simulink model "full_vehicle_sim"  (R2025b)
settings: Solver=VariableStepAuto  StartTime=0.0  StopTime=5  RelTol=1e-3
libraries: SimscapeFluids_lib x9, fl_lib x7, nesl_utility x5
(part 1 of 3)
settings Model: Creator=Owner  LastModifiedBy=25han
settings OptimizationCC: ReuseModelBlockBuffer=off
settings RTWCC: GPUComputeCapability=3.5

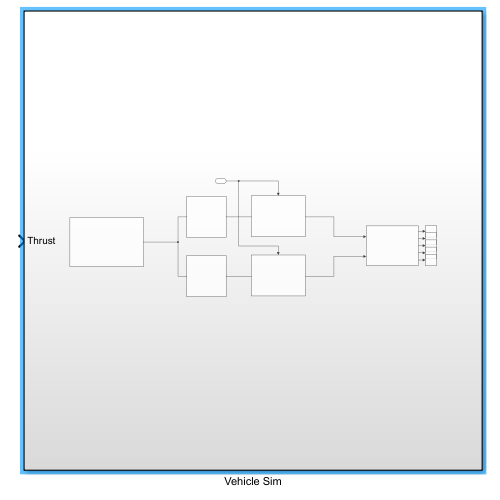
[thumbnail: Simulink's stored preview of the top-level diagram]
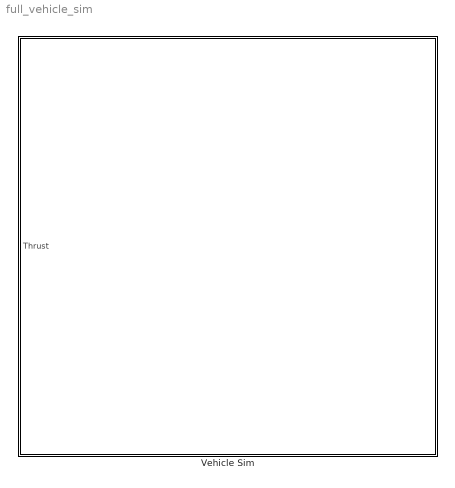
== system full_vehicle_sim ==
  Vehicle Sim : Subsystem

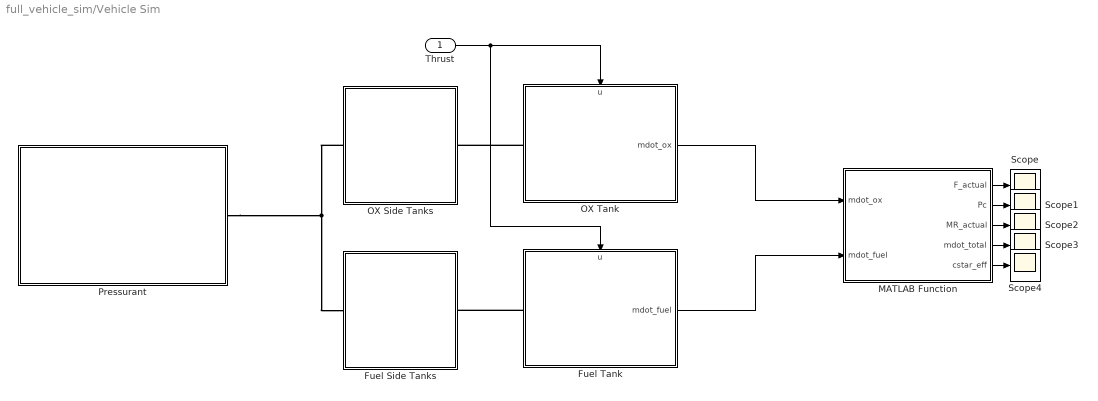
== system full_vehicle_sim/Vehicle Sim ==
  Thrust : Inport
  Fuel Side Tanks : Subsystem
  Fuel Tank : Subsystem
      settings: PortSchema="{\"entries\":[{\"content\":{\"sides\":[{\"content\":{\"connectorIds\":[\"LConn1\"]},\"type\":\"ConnectorPlacement.EquallySpacedRectSide\",\"uuid\":\"c996b4f4-0c8e-4748-a91d-4f7536df207c\"},{\"content\":{\"connectorIds\":[\"Out1\"],\"side\":\"RIGHT\"},\"type\":\"ConnectorPlacement.EquallySpacedRectSide\",\"uuid\":\"73da1da1-fc22-4773-8903-2723ce6ce475\"},{\"content\":{\"connectorIds\":[\"In1\"],\"side\":\"TOP\"},\"type\":\"ConnectorPlacement.EquallySpacedRectSide\",\"uuid\":\"cc756c5a-3437-4588-9c13-c05ccaf9d8e8\"}]},\"type\":\"ConnectorPlacement.EquallySpacedConnector\",\"uuid\":\"5391969f-ee8c-4c4c-8257-59a80b6e733b\"}],\"packageUris\":[\"http://schema.mathworks.com/mf0/Connector/R2020b\"],\"version\":\"1.0\"}"
  MATLAB Function : MATLAB Function  TreatAsAtomicUnit=on
  OX Side Tanks : Subsystem
  OX Tank : Subsystem
      settings: PortSchema="{\"entries\":[{\"content\":{\"sides\":[{\"content\":{\"connectorIds\":[\"LConn1\"]},\"type\":\"ConnectorPlacement.EquallySpacedRectSide\",\"uuid\":\"c996b4f4-0c8e-4748-a91d-4f7536df207c\"},{\"content\":{\"connectorIds\":[\"Out1\"],\"side\":\"RIGHT\"},\"type\":\"ConnectorPlacement.EquallySpacedRectSide\",\"uuid\":\"73da1da1-fc22-4773-8903-2723ce6ce475\"},{\"content\":{\"connectorIds\":[\"In1\"],\"side\":\"TOP\"},\"type\":\"ConnectorPlacement.EquallySpacedRectSide\",\"uuid\":\"cc756c5a-3437-4588-9c13-c05ccaf9d8e8\"}]},\"type\":\"ConnectorPlacement.EquallySpacedConnector\",\"uuid\":\"5391969f-ee8c-4c4c-8257-59a80b6e733b\"}],\"packageUris\":[\"http://schema.mathworks.com/mf0/Connector/R2020b\"],\"version\":\"1.0\"}"
  Pressurant : Subsystem
  Scope{,1..4} (5 alike) : Scope
      Scope settings: DataLoggingVariableName=ScopeData6
      Scope1 settings: DataLoggingVariableName=ScopeData7
      Scope2 settings: DataLoggingVariableName=ScopeData8
      Scope3 settings: DataLoggingVariableName=ScopeData9
      Scope4 settings: DataLoggingVariableName=ScopeData10
  wires:
  Thrust/1 -> OX Tank/1(u), Fuel Tank/1(u)
  Fuel Tank/1(mdot_fuel) -> MATLAB Function/2(mdot_fuel)
  OX Tank/1(mdot_ox) -> MATLAB Function/1(mdot_ox)
  MATLAB Function/2(Pc) -> Scope1/1
  MATLAB Function/3(MR_actual) -> Scope2/1
  MATLAB Function/4(mdot_total) -> Scope3/1
  MATLAB Function/5(cstar_eff) -> Scope4/1
  MATLAB Function/1(F_actual) -> Scope/1
  connections:
  OX Side Tanks/LConn1 -- Pressurant/RConn1 -- Fuel Side Tanks/LConn1
  OX Tank/LConn1 -- OX Side Tanks/RConn1
  Fuel Tank/LConn1 -- Fuel Side Tanks/RConn1

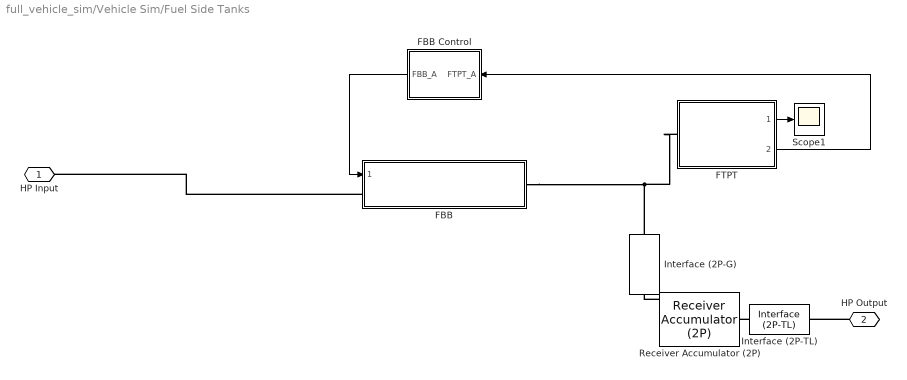
== system full_vehicle_sim/Vehicle Sim/Fuel Side Tanks ==
  FBB : Subsystem  ReferencedSubsystem=BangBang
  FBB Control : MATLAB Function  TreatAsAtomicUnit=on
  FTPT : Subsystem  ReferencedSubsystem=PT  max_press=5000  lower_val=4  upper_val=20
  Interface (2P-G) : SimscapeFluids_lib/Fluid Network Interfaces/Interface (2P-G)  area=0.01 m^2  vapor_error_spec=simscape.enum.assert.action.error
      settings: InternalSimscapePortConfiguration="{\"Bottom\":[],\"Left\":[{\"id\":\"x2P\",\"label\":\"2P\",\"type\":\"foundation.two_phase_fluid.two_phase_fluid\"}],\"Right\":[{\"id\":\"G\",\"label\":\"G\",\"type\":\"foundation.gas.gas\"}],\"Top\":[]}"
  Interface (2P-TL) : SimscapeFluids_lib/Fluid Network Interfaces/Interface (2P-TL)  area=0.01 m^2  liquid_error_spec=simscape.enum.assert.action.error
      settings: InternalSimscapePortConfiguration="{\"Bottom\":[],\"Left\":[{\"id\":\"x2P\",\"label\":\"2P\",\"type\":\"foundation.two_phase_fluid.two_phase_fluid\"}],\"Right\":[{\"id\":\"TL\",\"label\":\"TL\",\"type\":\"foundation.thermal_liquid.thermal_liquid\"}],\"Top\":[]}"
  Receiver Accumulator (2P) : SimscapeFluids_lib/Two-Phase Fluid/Tanks & Accumulators/Receiver Accumulator (2P)  volume=1 m^3  tank_area=0.5 m^2  area_AV=0.01 m^2  area_BV=0.01 m^2  area_AL=0.01 m^2  area_BL=0.01 m^2  V_frac_liq_error=simscape.enum.assert.action.none  V_frac_liq_min=0.05  V_frac_liq_max=0.95  V_frac_smooth=0.05  p_crit_error=simscape.enum.assert.action.error  hc_vap=20 W/(K*m^2)  hc_liq=100 W/(K*m^2)  p_init=0.101325 MPa  fraction_spec=fluids.two_phase_fluid.tanks_accumulators.enum.LiquidFractionSpec.Volume  M_frac_liq_init=0.5  V_frac_liq_init=0.5  saturated_init=true  energy_spec=fluids.two_phase_fluid.tanks_accumulators.enum.EnergySpec.SubcoolingSuperheating  delta_T_sub_init=5 deltaK  delta_T_sup_init=5 deltaK  T_liq_init=368.15 K  T_vap_init=378.15 K  h_liq_init=400 kJ/kg  h_vap_init=2700 kJ/kg  u_liq_init=400 kJ/kg  u_vap_init=2700 kJ/kg  tau_vap_cond=0.1 s
      settings: InternalSimscapePortConfiguration="{\"Bottom\":[],\"Left\":[{\"id\":\"AV\",\"label\":\"AV\",\"type\":\"foundation.two_phase_fluid.two_phase_fluid\"},{\"id\":\"AL\",\"label\":\"AL\",\"type\":\"foundation.two_phase_fluid.two_phase_fluid\"},{\"id\":\"H\",\"label\":\"H\",\"type\":\"foundation.thermal.thermal\"}],\"Right\":[{\"id\":\"BV\",\"label\":\"BV\",\"type\":\"foundation.two_phase_fluid.two_phase_fluid\"},{\"id\":\"BL\",\"label\":\"BL\",\"type\":\"foundation.two_phase_fluid.two_phase_fluid\"},{\"id\":\"L\",\"label\":\"L\",\"type\":\"output\"}],\"Top\":[]}"
  Scope1 : Scope
      settings: ActiveDisplayYMinimum=-330.96571  ActiveDisplayYMaximum=5077.33873
  HP Input : PMIOPort  Side=Left
  HP Output : PMIOPort  Port=2  Side=Right
  wires:
  FTPT/1 -> Scope1/1
  FTPT/2 -> FBB Control/1(FTPT_A)
  FBB Control/1(FBB_A) -> FBB/1
  connections:
  FBB/LConn1 -- HP Input/RConn1
  FTPT/LConn1 -- Interface (2P-G)/RConn1 -- FBB/RConn1
  Receiver Accumulator (2P)/LConn1 -- Interface (2P-G)/LConn1
  HP Output/RConn1 -- Interface (2P-TL)/RConn1
  Interface (2P-TL)/LConn1 -- Receiver Accumulator (2P)/RConn2

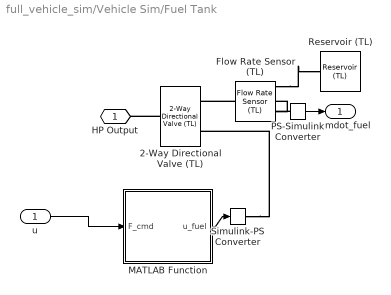
== system full_vehicle_sim/Vehicle Sim/Fuel Tank ==
  u : Inport
  2-Way Directional Valve (TL) : SimscapeFluids_lib/Thermal Liquid/Valves & Orifices/Directional Control Valves/2-Way Directional Valve (TL)  valve_spec=fluids.thermal_liquid.valves.directional_control_valves.enum.ValveSpec.Linear  S_max=5e-3 m  del_S_max=5e-3 m  area_max=1e-4 m^2  area_leak=1e-10 m^2  del_S_TLU=[0, .002, .004, .007, .017] m  valve_area_TLU=[1e-09, 2.0352e-07, 4.0736e-05, .00011438, .00034356] m^2  del_S_flow_TLU=[0, .002, .004, .007, .017] m  p_diff_TLU=[.3, .5, .7] MPa  vol_flow_TLU=1e-3 * [1.7e-05, 2e-05, 2.6e-05; .0035, .0045, .0053; .7, .9, 1.06; 1.96, 2.5, 3; 6, 7.7, 9.13] m^3/s  mdot_TLU=[1.7e-05, 2e-05, 2.6e-05; .0035, .0045, .0053; .7, .9, 1.06; 1.96, 2.5, 3; 6, 7.7, 9.13] kg/s  T_ref_in=293.15 K  p_ref_in=0.101325 MPa  Cd=0.64  Re_c=150  smoothing_factor=0.01  pressure_recovery=false  area=0.01 m^2
      settings: InternalSimscapePortConfiguration="{\"Bottom\":[],\"Left\":[{\"id\":\"A\",\"label\":\"A\",\"type\":\"foundation.thermal_liquid.thermal_liquid\"}],\"Right\":[{\"id\":\"S\",\"label\":\"S\",\"type\":\"input\"},{\"id\":\"B\",\"label\":\"B\",\"type\":\"foundation.thermal_liquid.thermal_liquid\"}],\"Top\":[]}"
  Flow Rate Sensor (TL) : fl_lib/Thermal Liquid/Sensors/Flow Rate Sensor (TL)  mass_flow_measure=true  volumetric_flow_measure=false  energy_flow_measure=true
      settings: InternalSimscapePortConfiguration="{\"Bottom\":[{\"id\":\"PHI\",\"label\":\"φ\",\"type\":\"output\"}],\"Left\":[{\"id\":\"A\",\"label\":\"A\",\"type\":\"foundation.thermal_liquid.thermal_liquid\"}],\"Right\":[{\"id\":\"B\",\"label\":\"B\",\"type\":\"foundation.thermal_liquid.thermal_liquid\"},{\"id\":\"M\",\"label\":\"M\",\"type\":\"output\"}],\"Top\":[]}"
  MATLAB Function : MATLAB Function  TreatAsAtomicUnit=on
  PS-Simulink Converter : nesl_utility/PS-Simulink Converter  PhysicalDomain=network_engine_domain  SubClassName=ps_output  LeftPortType=input  RightPortType=output  PseudoPeriodic=off  Frequencies=[]  VectorFormat=inherit  Unit=inherit  AffineConversion=off
  Reservoir (TL) : fl_lib/Thermal Liquid/Elements/Reservoir (TL)  pressure_spec=foundation.enum.pressure_spec.atmospheric  reservoir_pressure=0.101325 MPa  reservoir_temperature=293.15 K  area=0.01 m^2
  Simulink-PS Converter : nesl_utility/Simulink-PS Converter  PhysicalDomain=network_engine_domain  SubClassName=ps_input  LeftPortType=input  RightPortType=output  PseudoPeriodic=off  Frequencies=[]  NoiseDistribution=none  NoiseParameters=[]  Unit=1  AffineConversion=off  FilteringAndDerivatives=provide  SimscapeFilterOrder=1  InputFilterTimeConstant=0.001  UdotUserProvided=0
  HP Output : PMIOPort  Side=Left
  mdot_fuel : Outport
  wires:
  u/1 -> MATLAB Function/1(F_cmd)
  MATLAB Function/1(u_fuel) -> Simulink-PS Converter/1
  PS-Simulink Converter/1 -> mdot_fuel/1
  connections:
  2-Way Directional Valve (TL)/LConn1 -- HP Output/RConn1
  Flow Rate Sensor (TL)/LConn1 -- 2-Way Directional Valve (TL)/RConn2
  Simulink-PS Converter/RConn1 -- 2-Way Directional Valve (TL)/RConn1
  PS-Simulink Converter/LConn1 -- Flow Rate Sensor (TL)/RConn2
  Flow Rate Sensor (TL)/RConn1 -- Reservoir (TL)/LConn1

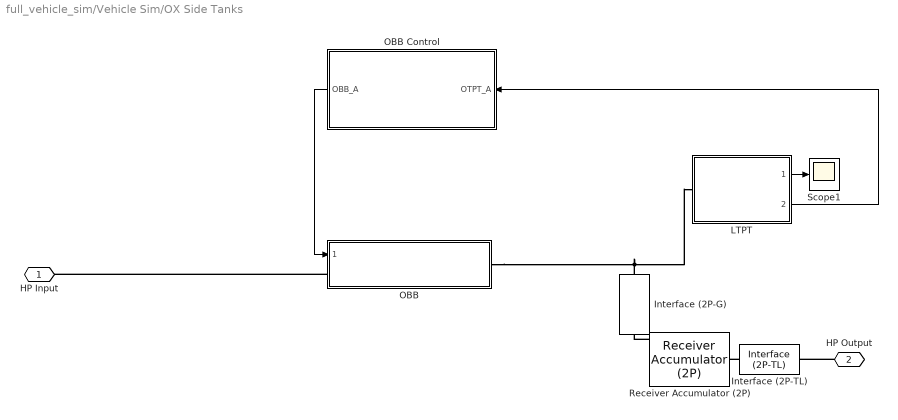
== system full_vehicle_sim/Vehicle Sim/OX Side Tanks ==
  Interface (2P-G) : SimscapeFluids_lib/Fluid Network Interfaces/Interface (2P-G)  area=0.01 m^2  vapor_error_spec=simscape.enum.assert.action.error
      settings: InternalSimscapePortConfiguration="{\"Bottom\":[],\"Left\":[{\"id\":\"x2P\",\"label\":\"2P\",\"type\":\"foundation.two_phase_fluid.two_phase_fluid\"}],\"Right\":[{\"id\":\"G\",\"label\":\"G\",\"type\":\"foundation.gas.gas\"}],\"Top\":[]}"
  Interface (2P-TL) : SimscapeFluids_lib/Fluid Network Interfaces/Interface (2P-TL)  area=0.01 m^2  liquid_error_spec=simscape.enum.assert.action.error
      settings: InternalSimscapePortConfiguration="{\"Bottom\":[],\"Left\":[{\"id\":\"x2P\",\"label\":\"2P\",\"type\":\"foundation.two_phase_fluid.two_phase_fluid\"}],\"Right\":[{\"id\":\"TL\",\"label\":\"TL\",\"type\":\"foundation.thermal_liquid.thermal_liquid\"}],\"Top\":[]}"
  LTPT : Subsystem  ReferencedSubsystem=PT  max_press=5000  lower_val=4  upper_val=20
  OBB : Subsystem  ReferencedSubsystem=BangBang
  OBB Control : MATLAB Function  TreatAsAtomicUnit=on
  Receiver Accumulator (2P) : SimscapeFluids_lib/Two-Phase Fluid/Tanks & Accumulators/Receiver Accumulator (2P)  volume=1 m^3  tank_area=0.5 m^2  area_AV=0.01 m^2  area_BV=0.01 m^2  area_AL=0.01 m^2  area_BL=0.01 m^2  V_frac_liq_error=simscape.enum.assert.action.none  V_frac_liq_min=0.05  V_frac_liq_max=0.95  V_frac_smooth=0.05  p_crit_error=simscape.enum.assert.action.error  hc_vap=20 W/(K*m^2)  hc_liq=100 W/(K*m^2)  p_init=0.101325 MPa  fraction_spec=fluids.two_phase_fluid.tanks_accumulators.enum.LiquidFractionSpec.Volume  M_frac_liq_init=0.5  V_frac_liq_init=0.5  saturated_init=true  energy_spec=fluids.two_phase_fluid.tanks_accumulators.enum.EnergySpec.SubcoolingSuperheating  delta_T_sub_init=5 deltaK  delta_T_sup_init=5 deltaK  T_liq_init=368.15 K  T_vap_init=378.15 K  h_liq_init=400 kJ/kg  h_vap_init=2700 kJ/kg  u_liq_init=400 kJ/kg  u_vap_init=2700 kJ/kg  tau_vap_cond=0.1 s
      settings: InternalSimscapePortConfiguration="{\"Bottom\":[],\"Left\":[{\"id\":\"AV\",\"label\":\"AV\",\"type\":\"foundation.two_phase_fluid.two_phase_fluid\"},{\"id\":\"AL\",\"label\":\"AL\",\"type\":\"foundation.two_phase_fluid.two_phase_fluid\"},{\"id\":\"H\",\"label\":\"H\",\"type\":\"foundation.thermal.thermal\"}],\"Right\":[{\"id\":\"BV\",\"label\":\"BV\",\"type\":\"foundation.two_phase_fluid.two_phase_fluid\"},{\"id\":\"BL\",\"label\":\"BL\",\"type\":\"foundation.two_phase_fluid.two_phase_fluid\"},{\"id\":\"L\",\"label\":\"L\",\"type\":\"output\"}],\"Top\":[]}"
  Scope1 : Scope
      settings: ActiveDisplayYMinimum=-330.96571  ActiveDisplayYMaximum=5077.33873
  HP Input : PMIOPort  Side=Left
  HP Output : PMIOPort  Port=2  Side=Right
  wires:
  LTPT/1 -> Scope1/1
  OBB Control/1(OBB_A) -> OBB/1
  LTPT/2 -> OBB Control/1(OTPT_A)
  connections:
  OBB/LConn1 -- HP Input/RConn1
  OBB/RConn1 -- Interface (2P-G)/RConn1 -- LTPT/LConn1
  Receiver Accumulator (2P)/LConn1 -- Interface (2P-G)/LConn1
  HP Output/RConn1 -- Interface (2P-TL)/RConn1
  Interface (2P-TL)/LConn1 -- Receiver Accumulator (2P)/RConn2

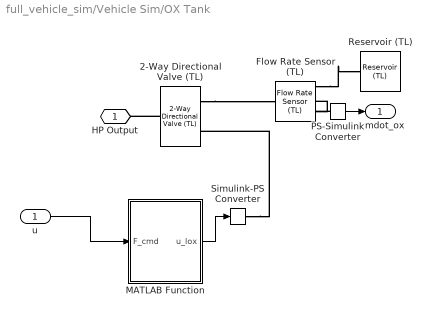
== system full_vehicle_sim/Vehicle Sim/OX Tank ==
  u : Inport
  2-Way Directional Valve (TL) : SimscapeFluids_lib/Thermal Liquid/Valves & Orifices/Directional Control Valves/2-Way Directional Valve (TL)  valve_spec=fluids.thermal_liquid.valves.directional_control_valves.enum.ValveSpec.Linear  S_max=5e-3 m  del_S_max=5e-3 m  area_max=1e-4 m^2  area_leak=1e-10 m^2  del_S_TLU=[0, .002, .004, .007, .017] m  valve_area_TLU=[1e-09, 2.0352e-07, 4.0736e-05, .00011438, .00034356] m^2  del_S_flow_TLU=[0, .002, .004, .007, .017] m  p_diff_TLU=[.3, .5, .7] MPa  vol_flow_TLU=1e-3 * [1.7e-05, 2e-05, 2.6e-05; .0035, .0045, .0053; .7, .9, 1.06; 1.96, 2.5, 3; 6, 7.7, 9.13] m^3/s  mdot_TLU=[1.7e-05, 2e-05, 2.6e-05; .0035, .0045, .0053; .7, .9, 1.06; 1.96, 2.5, 3; 6, 7.7, 9.13] kg/s  T_ref_in=293.15 K  p_ref_in=0.101325 MPa  Cd=0.64  Re_c=150  smoothing_factor=0.01  pressure_recovery=false  area=0.01 m^2
      settings: InternalSimscapePortConfiguration="{\"Bottom\":[],\"Left\":[{\"id\":\"A\",\"label\":\"A\",\"type\":\"foundation.thermal_liquid.thermal_liquid\"}],\"Right\":[{\"id\":\"S\",\"label\":\"S\",\"type\":\"input\"},{\"id\":\"B\",\"label\":\"B\",\"type\":\"foundation.thermal_liquid.thermal_liquid\"}],\"Top\":[]}"
  Flow Rate Sensor (TL) : fl_lib/Thermal Liquid/Sensors/Flow Rate Sensor (TL)  mass_flow_measure=true  volumetric_flow_measure=false  energy_flow_measure=true
      settings: InternalSimscapePortConfiguration="{\"Bottom\":[{\"id\":\"PHI\",\"label\":\"φ\",\"type\":\"output\"}],\"Left\":[{\"id\":\"A\",\"label\":\"A\",\"type\":\"foundation.thermal_liquid.thermal_liquid\"}],\"Right\":[{\"id\":\"B\",\"label\":\"B\",\"type\":\"foundation.thermal_liquid.thermal_liquid\"},{\"id\":\"M\",\"label\":\"M\",\"type\":\"output\"}],\"Top\":[]}"
  MATLAB Function : MATLAB Function  TreatAsAtomicUnit=on
  PS-Simulink Converter : nesl_utility/PS-Simulink Converter  PhysicalDomain=network_engine_domain  SubClassName=ps_output  LeftPortType=input  RightPortType=output  PseudoPeriodic=off  Frequencies=[]  VectorFormat=inherit  Unit=inherit  AffineConversion=off
  Reservoir (TL) : fl_lib/Thermal Liquid/Elements/Reservoir (TL)  pressure_spec=foundation.enum.pressure_spec.atmospheric  reservoir_pressure=0.101325 MPa  reservoir_temperature=293.15 K  area=0.01 m^2
  Simulink-PS Converter : nesl_utility/Simulink-PS Converter  PhysicalDomain=network_engine_domain  SubClassName=ps_input  LeftPortType=input  RightPortType=output  PseudoPeriodic=off  Frequencies=[]  NoiseDistribution=none  NoiseParameters=[]  Unit=1  AffineConversion=off  FilteringAndDerivatives=provide  SimscapeFilterOrder=1  InputFilterTimeConstant=0.001  UdotUserProvided=0
  HP Output : PMIOPort  Side=Left
  mdot_ox : Outport
  wires:
  u/1 -> MATLAB Function/1(F_cmd)
  MATLAB Function/1(u_lox) -> Simulink-PS Converter/1
  PS-Simulink Converter/1 -> mdot_ox/1
  connections:
  2-Way Directional Valve (TL)/LConn1 -- HP Output/RConn1
  Simulink-PS Converter/RConn1 -- 2-Way Directional Valve (TL)/RConn1
  2-Way Directional Valve (TL)/RConn2 -- Flow Rate Sensor (TL)/LConn1
  PS-Simulink Converter/LConn1 -- Flow Rate Sensor (TL)/RConn2
  Flow Rate Sensor (TL)/RConn1 -- Reservoir (TL)/LConn1
